simulink model "GA_driveline_Gear_19a"  (R2019a)
settings: Solver=ode23t  StartTime=0.0  StopTime=1  MaxStep=1e-2  RelTol=1e-3  AbsTol=1e-3  EnableMultiTasking=on
StopFcn:
  | GA_plot
libraries: fl_lib x29, nesl_utility x20, sdl_lib x4
CloseFcn:
  | try,close(h1_sdl_gear_backlash),end
  | clear h1_sdl_gear_backlash
  | 
  | 
  | clear simlog_sdl_gear_backlash
Description:
  | Gear with Backlash
settings Model: FPTRunName=Active  ExtModeAutoUpdateStatusClock=off  Creator=MathWorks  LastModifiedBy=JPark
settings SolverCC: AutoScaleAbsTol=off
settings DataIOCC: MaxDataPoints=10000  SaveFormat=Array  SignalLoggingSaveFormat=ModelDataLogs  SaveOutput=off  SignalLogging=off  DSMLogging=off  ReturnWorkspaceOutputs=off  SignalLoggingName=logsout_sdl_gear_backlash
settings OptimizationCC: ExpressionDepthLimit=2147483647  InitFltsAndDblsToZero=on  LifeSpan=inf
settings DebuggingCC: AlgebraicLoopMsg=none  SaveWithParameterizedLinksMsg=none  SignalResolutionControl=TryResolveAllWithWarning  MultiTaskDSMMsg=warning  MultiTaskCondExecSysMsg=none  SigSpecEnsureSampleTimeMsg=none  StateNameClashWarn=warning  SFUnexpectedBacktrackingDiag=warning  SFNoUnconditionalDefaultTransitionDiag=warning  SFExecutionAtInitializationDiag=none  ArithmeticOperatorsInVariantConditions=warning
settings HardwareCC: ProdBitPerPointer=32  ProdBitPerSizeT=32  ProdBitPerPtrDiffT=32  ProdLargestAtomicFloat=None  ProdIntDivRoundTo=Undefined  ProdEndianess=Unspecified  ProdWordSize=32  ProdHWDeviceType=32-bit Generic  TargetBitPerPointer=64  TargetBitPerSizeT=64  TargetBitPerPtrDiffT=64  TargetLongLongMode=on  TargetIntDivRoundTo=Zero  TargetEndianess=LittleEndian  TargetWordSize=64  TargetHWDeviceType=MATLAB Host  ProdEqTarget=off
settings ModelReferenceCC: PropagateSignalLabelsOutOfModel=off
settings SFSimCC: SimUseLocalCustomCode=off
settings RTWCC: Description=Generic Real-Time Target  RTWUseLocalCustomCode=off
settings CodeAppCC: StateflowObjectComments=on
settings GRTTargetCC: TargetLangStandard=C89/C90 (ANSI)  GeneratePreprocessorConditionals=Disable all  CombineOutputUpdateFcns=off  GRTInterface=on
settings ConfigComp: CovMetricSettings=dw  CovHtmlReporting=on  CovSaveCumulativeToWorkspaceVar=on  CovSaveSingleToWorkspaceVar=on  CovShowResultsExplorer=off  CovExternalEMLEnable=off
settings SimscapeCC: SimscapeLogType=all  SimscapeLogSimulationStatistics=on  SimscapeLogName=simlog_sdl_gear_backlash  SimscapeLogLimitData=off  SimscapeLogDataHistory=15000

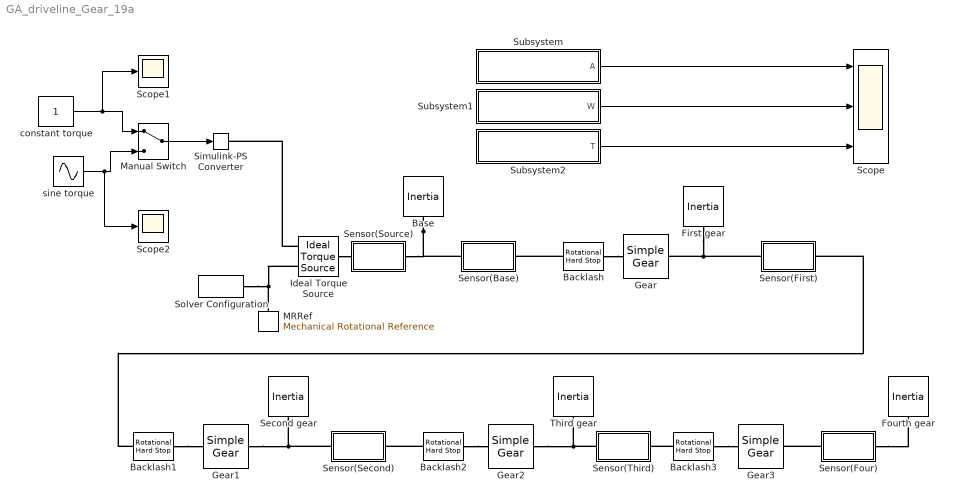
== system GA_driveline_Gear_19a ==
  Backlash{,1..3} (4 alike) : fl_lib/Mechanical/Rotational Elements/Rotational Hard Stop  upper_bnd=0.2 deg  lower_bnd=-0.2 deg  stiff_up=1e+6 N*m/rad  stiff_low=1e+6 N*m/rad  D_up=100 N*m/(rad/s)  D_low=100 N*m/(rad/s)  model=simscape.enum.hardstop.fulldamped  transition=0.001 rad  w_specify=off  w_priority=None  w=0 rad/s  w_nominal_specify=off  w_nominal_unit=rad/s  w_nominal_value=1  t_specify=off  t_priority=None  t=0 N*m  t_nominal_specify=off  t_nominal_unit=N*m  t_nominal_value=1  phi_specify=on  phi_priority=High  phi=0 rad  phi_nominal_specify=off  phi_nominal_unit=rad  phi_nominal_value=1
      settings: SourceProductName=Simscape  SourceProductBaseCode=SS
  Base : fl_lib/Mechanical/Rotational Elements/Inertia  inertia=1 kg*m^2  w_specify=on  w_priority=High  w=0 rad/s  w_nominal_specify=off  w_nominal_unit=rad/s  w_nominal_value=1  t_specify=off  t_priority=None  t=0 N*m  t_nominal_specify=off  t_nominal_unit=N*m  t_nominal_value=1
  First gear : fl_lib/Mechanical/Rotational Elements/Inertia  inertia=1 kg*m^2  w_specify=on  w_priority=High  w=0 rad/s  w_nominal_specify=off  w_nominal_unit=rad/s  w_nominal_value=1  t_specify=off  t_priority=None  t=0 N*m  t_nominal_specify=off  t_nominal_unit=N*m  t_nominal_value=1
  Fourth gear : fl_lib/Mechanical/Rotational Elements/Inertia  inertia=2e-5 kg*m^2  w_specify=on  w_priority=High  w=0 rad/s  w_nominal_specify=off  w_nominal_unit=rad/s  w_nominal_value=1  t_specify=off  t_priority=None  t=0 N*m  t_nominal_specify=off  t_nominal_unit=N*m  t_nominal_value=1
  Gear : sdl_lib/Gears/Simple Gear  ratio=4.5  rotation_direction=1  friction_model=sdl.enum.gear_efficiencies_load.off  T_noload=0.1 N*m  T_nom=5 N*m  efficiency_nom=0.8  efficiency=0.8  mu_visc=[ 0 0 ] N*m/(rad/s)  w_thr=0.01 rad/s  pwr_thr=0.001 W  enable_faults=simscape.enum.onoff.off  efficiency_fault=0.05  external_fault=simscape.enum.onoff.off  temporal_fault=simscape.enum.onoff.off  fault_time=5 s  fault_angles=pi / 12 rad  report_fault=1  temperature_TLU=[ 280 300 320 ] K  load_TLU=[ 1 5 10 ] N*m  efficiency_TLU=[ 0.95 0.9 0.85 ]  efficiency_TLU2=[ 0.85 0.8 0.75; 0.95 0.9 0.85; 0.85 0.8 0.7 ]  thermal_mass=50 J/K  T_init=300 K
      settings: SourceProductName=Simscape Driveline
  Gear1 : sdl_lib/Gears/Simple Gear  ratio=4.5  rotation_direction=1  friction_model=sdl.enum.gear_efficiencies_load.off  T_noload=0.1 N*m  T_nom=5 N*m  efficiency_nom=0.8  efficiency=0.8  mu_visc=[ 0 0 ] N*m/(rad/s)  w_thr=0.01 rad/s  pwr_thr=0.001 W  enable_faults=simscape.enum.onoff.off  efficiency_fault=0.05  external_fault=simscape.enum.onoff.off  temporal_fault=simscape.enum.onoff.off  fault_time=5 s  fault_angles=pi / 12 rad  report_fault=1  temperature_TLU=[ 280 300 320 ] K  load_TLU=[ 1 5 10 ] N*m  efficiency_TLU=[ 0.95 0.9 0.85 ]  efficiency_TLU2=[ 0.85 0.8 0.75; 0.95 0.9 0.85; 0.85 0.8 0.7 ]  thermal_mass=50 J/K  T_init=300 K
      settings: SourceProductName=Simscape Driveline
  Gear2 : sdl_lib/Gears/Simple Gear  ratio=4.5  rotation_direction=1  friction_model=sdl.enum.gear_efficiencies_load.off  T_noload=0.1 N*m  T_nom=5 N*m  efficiency_nom=0.8  efficiency=0.8  mu_visc=[ 0 0 ] N*m/(rad/s)  w_thr=0.01 rad/s  pwr_thr=0.001 W  enable_faults=simscape.enum.onoff.off  efficiency_fault=0.05  external_fault=simscape.enum.onoff.off  temporal_fault=simscape.enum.onoff.off  fault_time=5 s  fault_angles=pi / 12 rad  report_fault=1  temperature_TLU=[ 280 300 320 ] K  load_TLU=[ 1 5 10 ] N*m  efficiency_TLU=[ 0.95 0.9 0.85 ]  efficiency_TLU2=[ 0.85 0.8 0.75; 0.95 0.9 0.85; 0.85 0.8 0.7 ]  thermal_mass=50 J/K  T_init=300 K
      settings: SourceProductName=Simscape Driveline
  Gear3 : sdl_lib/Gears/Simple Gear  ratio=3.1  rotation_direction=1  friction_model=sdl.enum.gear_efficiencies_load.off  T_noload=0.1 N*m  T_nom=5 N*m  efficiency_nom=0.8  efficiency=0.8  mu_visc=[ 0 0 ] N*m/(rad/s)  w_thr=0.01 rad/s  pwr_thr=0.001 W  enable_faults=simscape.enum.onoff.off  efficiency_fault=0.05  external_fault=simscape.enum.onoff.off  temporal_fault=simscape.enum.onoff.off  fault_time=5 s  fault_angles=pi / 12 rad  report_fault=1  temperature_TLU=[ 280 300 320 ] K  load_TLU=[ 1 5 10 ] N*m  efficiency_TLU=[ 0.95 0.9 0.85 ]  efficiency_TLU2=[ 0.85 0.8 0.75; 0.95 0.9 0.85; 0.85 0.8 0.7 ]  thermal_mass=50 J/K  T_init=300 K
      settings: SourceProductName=Simscape Driveline
  Ideal Torque Source : fl_lib/Mechanical/Mechanical Sources/Ideal Torque Source
  MRRef : fl_lib/Mechanical/Rotational Elements/Mechanical Rotational Reference
  Manual Switch : ManualSwitch
  Scope : Scope  NumInputPorts=3
  Scope1 : Scope
  Scope2 : Scope
  Second gear : fl_lib/Mechanical/Rotational Elements/Inertia  inertia=1 kg*m^2  w_specify=on  w_priority=High  w=0 rad/s  w_nominal_specify=off  w_nominal_unit=rad/s  w_nominal_value=1  t_specify=off  t_priority=None  t=0 N*m  t_nominal_specify=off  t_nominal_unit=N*m  t_nominal_value=1
  Sensor(Base) : Subsystem
  Sensor(First) : Subsystem
  Sensor(Four) : Subsystem
  Sensor(Second) : Subsystem
  Sensor(Source) : Subsystem
  Sensor(Third) : Subsystem
  Simulink-PS Converter : nesl_utility/Simulink-PS Converter  PhysicalDomain=network_engine_domain  SubClassName=ps_input  LeftPortType=input  RightPortType=output  PseudoPeriodic=off  Frequencies=[]  NoiseDistribution=none  NoiseParameters=[]  Unit=1  AffineConversion=off  FilteringAndDerivatives=provide  SimscapeFilterOrder=1  InputFilterTimeConstant=0.001  UdotUserProvided=0
  Solver Configuration : nesl_utility/Solver Configuration  PhysicalDomain=network_engine_domain  SubClassName=solver  LeftPortType=input  RightPortType=generic  Tones=[]  Harmonics=[]  SimulateNoise=off  Profile=off  UseLocalSampling=off  EnableSwitchedLinearOptims=on  FrequencyDomain=off  UseCCode=off  RelTol=0.001  AbsTol=1e-06  MinStep=1e-09  ToWorkspace=off  RevertToSquareIcSolve=off  NumHomotopyIterations=100  PhasorMode=off  PhasorModeNumHarmonics=1  DoDC=off  ResidualTolerance=1e-9  UseLocalSolver=off  LocalSolverChoice=NE_PARTITIONING_ADVANCER  LocalSolverSampleTime=0.0001  DoFixedCost=off  MaxNonlinIter=3  MaxModeIter=2  LinearAlgebra=auto  EquationFormulation=NE_TIME_EF  DelaysMemoryBudget=1024  AutomaticFiltering=on  FilteringTimeConstant=0.001  PartitionStorageMethod=EXHAUSTIVE  PartitionMemoryBudget=1024  PartitionMethod=ROBUST
  Subsystem : Subsystem
  Subsystem1 : Subsystem
  Subsystem2 : Subsystem
  Third gear : fl_lib/Mechanical/Rotational Elements/Inertia  inertia=1 kg*m^2  w_specify=on  w_priority=High  w=0 rad/s  w_nominal_specify=off  w_nominal_unit=rad/s  w_nominal_value=1  t_specify=off  t_priority=None  t=0 N*m  t_nominal_specify=off  t_nominal_unit=N*m  t_nominal_value=1
  constant torque : Constant
  sine torque : Sin  Amplitude=100  Frequency=2*pi*1  Phase=1/2*pi  SampleTime=0
  wires:
  constant torque/1 -> Scope1/1, Manual Switch/1
  sine torque/1 -> Scope2/1, Manual Switch/2
  Manual Switch/1 -> Simulink-PS Converter/1
  Subsystem/1(A) -> Scope/1
  Subsystem1/1(W) -> Scope/2
  Subsystem2/1(T) -> Scope/3
  connections:
  Base/LConn1 -- Sensor(Source)/RConn1 -- Sensor(Base)/LConn1
  MRRef/LConn1 -- Ideal Torque Source/RConn2 -- Solver Configuration/RConn1
  Backlash/RConn1 -- Gear/LConn1
  First gear/LConn1 -- Sensor(First)/LConn1 -- Gear/RConn1
  Backlash1/RConn1 -- Gear1/LConn1
  Gear1/RConn1 -- Sensor(Second)/LConn1 -- Second gear/LConn1
  Gear2/RConn1 -- Sensor(Third)/LConn1 -- Third gear/LConn1
  Backlash2/RConn1 -- Gear2/LConn1
  Backlash3/RConn1 -- Gear3/LConn1
  Ideal Torque Source/RConn1 -- Simulink-PS Converter/RConn1
  Backlash/LConn1 -- Sensor(Base)/RConn1
  Backlash1/LConn1 -- Sensor(First)/RConn1
  Backlash2/LConn1 -- Sensor(Second)/RConn1
  Backlash3/LConn1 -- Sensor(Third)/RConn1
  Sensor(Four)/LConn1 -- Gear3/RConn1
  Sensor(Four)/RConn1 -- Fourth gear/LConn1
  Ideal Torque Source/LConn1 -- Sensor(Source)/LConn1

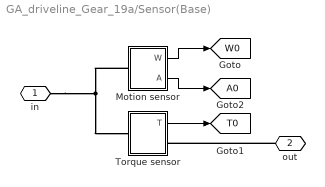
== system GA_driveline_Gear_19a/Sensor(Base) ==
  Motion sensor : Subsystem
  Torque sensor : Subsystem
  in : PMIOPort  Side=Left
  out : PMIOPort  Port=2  Side=Right
  tag scope: A0=global, T0=global, W0=global
  wires:
  Motion sensor/1(W) -> [W0]
  Torque sensor/1(T) -> [T0]
  Motion sensor/2(A) -> [A0]
  connections:
  in/RConn1 -- Motion sensor/LConn1 -- Torque sensor/LConn1
  out/RConn1 -- Torque sensor/RConn1

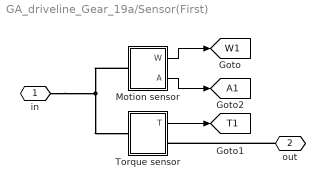
== system GA_driveline_Gear_19a/Sensor(First) ==
  Motion sensor : Subsystem
  Torque sensor : Subsystem
  in : PMIOPort  Side=Left
  out : PMIOPort  Port=2  Side=Right
  tag scope: A1=global, T1=global, W1=global
  wires:
  Motion sensor/1(W) -> [W1]
  Torque sensor/1(T) -> [T1]
  Motion sensor/2(A) -> [A1]
  connections:
  in/RConn1 -- Motion sensor/LConn1 -- Torque sensor/LConn1
  out/RConn1 -- Torque sensor/RConn1

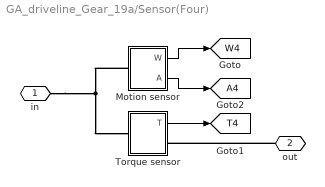
== system GA_driveline_Gear_19a/Sensor(Four) ==
  Motion sensor : Subsystem
  Torque sensor : Subsystem
  in : PMIOPort  Side=Left
  out : PMIOPort  Port=2  Side=Right
  tag scope: A4=global, T4=global, W4=global
  wires:
  Motion sensor/1(W) -> [W4]
  Torque sensor/1(T) -> [T4]
  Motion sensor/2(A) -> [A4]
  connections:
  in/RConn1 -- Motion sensor/LConn1 -- Torque sensor/LConn1
  out/RConn1 -- Torque sensor/RConn1

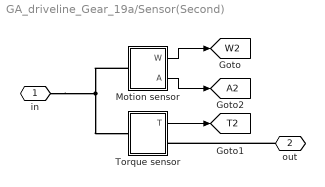
== system GA_driveline_Gear_19a/Sensor(Second) ==
  Motion sensor : Subsystem
  Torque sensor : Subsystem
  in : PMIOPort  Side=Left
  out : PMIOPort  Port=2  Side=Right
  tag scope: A2=global, T2=global, W2=global
  wires:
  Motion sensor/1(W) -> [W2]
  Torque sensor/1(T) -> [T2]
  Motion sensor/2(A) -> [A2]
  connections:
  in/RConn1 -- Motion sensor/LConn1 -- Torque sensor/LConn1
  out/RConn1 -- Torque sensor/RConn1

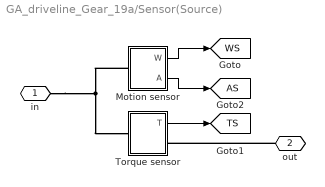
== system GA_driveline_Gear_19a/Sensor(Source) ==
  Motion sensor : Subsystem
  Torque sensor : Subsystem
  in : PMIOPort  Side=Left
  out : PMIOPort  Port=2  Side=Right
  tag scope: AS=global, TS=global, WS=global
  wires:
  Motion sensor/1(W) -> [WS]
  Torque sensor/1(T) -> [TS]
  Motion sensor/2(A) -> [AS]
  connections:
  in/RConn1 -- Motion sensor/LConn1 -- Torque sensor/LConn1
  out/RConn1 -- Torque sensor/RConn1

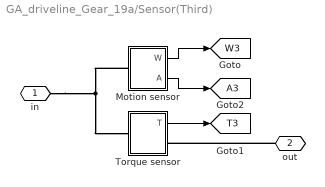
== system GA_driveline_Gear_19a/Sensor(Third) ==
  Motion sensor : Subsystem
  Torque sensor : Subsystem
  in : PMIOPort  Side=Left
  out : PMIOPort  Port=2  Side=Right
  tag scope: A3=global, T3=global, W3=global
  wires:
  Motion sensor/1(W) -> [W3]
  Torque sensor/1(T) -> [T3]
  Motion sensor/2(A) -> [A3]
  connections:
  in/RConn1 -- Motion sensor/LConn1 -- Torque sensor/LConn1
  out/RConn1 -- Torque sensor/RConn1

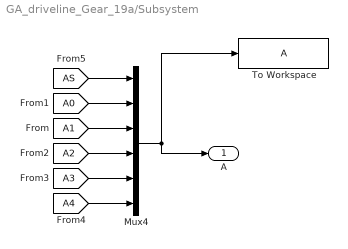
== system GA_driveline_Gear_19a/Subsystem ==
  Mux4 : Mux  Inputs=6
  To Workspace : ToWorkspace  VariableName=A  SaveFormat=Timeseries  SampleTime=-1
  A : Outport
  wires:
  Mux4/1 -> A/1, To Workspace/1
  [AS] -> Mux4/1
  [A0] -> Mux4/2
  [A1] -> Mux4/3
  [A2] -> Mux4/4
  [A3] -> Mux4/5
  [A4] -> Mux4/6

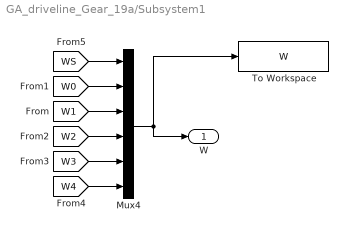
== system GA_driveline_Gear_19a/Subsystem1 ==
  Mux4 : Mux  Inputs=6
  To Workspace : ToWorkspace  VariableName=W  SaveFormat=Timeseries  SampleTime=-1
  W : Outport
  wires:
  Mux4/1 -> W/1, To Workspace/1
  [WS] -> Mux4/1
  [W0] -> Mux4/2
  [W1] -> Mux4/3
  [W2] -> Mux4/4
  [W3] -> Mux4/5
  [W4] -> Mux4/6

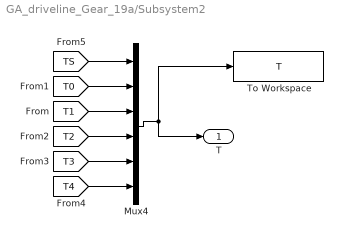
== system GA_driveline_Gear_19a/Subsystem2 ==
  Mux4 : Mux  Inputs=6
  To Workspace : ToWorkspace  VariableName=T  SaveFormat=Timeseries  SampleTime=-1
  T : Outport
  wires:
  Mux4/1 -> T/1, To Workspace/1
  [TS] -> Mux4/1
  [T0] -> Mux4/2
  [T1] -> Mux4/3
  [T2] -> Mux4/4
  [T3] -> Mux4/5
  [T4] -> Mux4/6

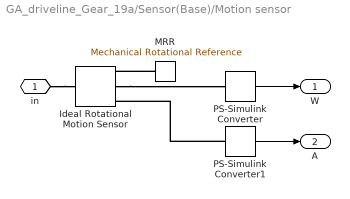
== system GA_driveline_Gear_19a/Sensor(Base)/Motion sensor ==
  Ideal Rotational Motion Sensor : fl_lib/Mechanical/Mechanical Sensors/Ideal Rotational Motion Sensor  offset=0 rad
  MRR : fl_lib/Mechanical/Rotational Elements/Mechanical Rotational Reference
  PS-Simulink Converter : nesl_utility/PS-Simulink Converter  PhysicalDomain=network_engine_domain  SubClassName=ps_output  LeftPortType=input  RightPortType=output  PseudoPeriodic=off  Frequencies=[]  Unit=rad/s  AffineConversion=off
  PS-Simulink Converter1 : nesl_utility/PS-Simulink Converter  PhysicalDomain=network_engine_domain  SubClassName=ps_output  LeftPortType=input  RightPortType=output  PseudoPeriodic=off  Frequencies=[]  Unit=rad  AffineConversion=off
  in : PMIOPort  Side=Left
  W : Outport  VectorParamsAs1DForOutWhenUnconnected=off
  A : Outport  Port=2  VectorParamsAs1DForOutWhenUnconnected=off
  wires:
  PS-Simulink Converter/1 -> W/1
  PS-Simulink Converter1/1 -> A/1
  connections:
  in/RConn1 -- Ideal Rotational Motion Sensor/LConn1
  Ideal Rotational Motion Sensor/RConn2 -- PS-Simulink Converter/LConn1
  MRR/LConn1 -- Ideal Rotational Motion Sensor/RConn1
  PS-Simulink Converter1/LConn1 -- Ideal Rotational Motion Sensor/RConn3

== system GA_driveline_Gear_19a/Sensor(Base)/Torque sensor ==
  PS2S : nesl_utility/PS-Simulink Converter  PhysicalDomain=network_engine_domain  SubClassName=ps_output  LeftPortType=input  RightPortType=output  PseudoPeriodic=off  Frequencies=[]  Unit=N*m  AffineConversion=off
  Torque Sensor : fl_lib/Mechanical/Mechanical Sensors/Ideal Torque Sensor
  B : PMIOPort  Side=Right
  in : PMIOPort  Port=2  Side=Left
  T : Outport  VectorParamsAs1DForOutWhenUnconnected=off
  wires:
  PS2S/1 -> T/1
  connections:
  in/RConn1 -- Torque Sensor/LConn1
  B/RConn1 -- Torque Sensor/RConn1
  Torque Sensor/RConn2 -- PS2S/LConn1

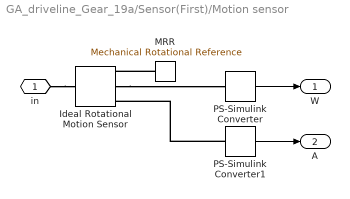
== system GA_driveline_Gear_19a/Sensor(First)/Motion sensor ==
  Ideal Rotational Motion Sensor : fl_lib/Mechanical/Mechanical Sensors/Ideal Rotational Motion Sensor  offset=0 rad
  MRR : fl_lib/Mechanical/Rotational Elements/Mechanical Rotational Reference
  PS-Simulink Converter : nesl_utility/PS-Simulink Converter  PhysicalDomain=network_engine_domain  SubClassName=ps_output  LeftPortType=input  RightPortType=output  PseudoPeriodic=off  Frequencies=[]  Unit=rad/s  AffineConversion=off
  PS-Simulink Converter1 : nesl_utility/PS-Simulink Converter  PhysicalDomain=network_engine_domain  SubClassName=ps_output  LeftPortType=input  RightPortType=output  PseudoPeriodic=off  Frequencies=[]  Unit=rad  AffineConversion=off
  in : PMIOPort  Side=Left
  W : Outport  VectorParamsAs1DForOutWhenUnconnected=off
  A : Outport  Port=2  VectorParamsAs1DForOutWhenUnconnected=off
  wires:
  PS-Simulink Converter/1 -> W/1
  PS-Simulink Converter1/1 -> A/1
  connections:
  in/RConn1 -- Ideal Rotational Motion Sensor/LConn1
  Ideal Rotational Motion Sensor/RConn2 -- PS-Simulink Converter/LConn1
  MRR/LConn1 -- Ideal Rotational Motion Sensor/RConn1
  PS-Simulink Converter1/LConn1 -- Ideal Rotational Motion Sensor/RConn3

== system GA_driveline_Gear_19a/Sensor(First)/Torque sensor ==
  PS2S : nesl_utility/PS-Simulink Converter  PhysicalDomain=network_engine_domain  SubClassName=ps_output  LeftPortType=input  RightPortType=output  PseudoPeriodic=off  Frequencies=[]  Unit=N*m  AffineConversion=off
  Torque Sensor : fl_lib/Mechanical/Mechanical Sensors/Ideal Torque Sensor
  B : PMIOPort  Side=Right
  in : PMIOPort  Port=2  Side=Left
  T : Outport  VectorParamsAs1DForOutWhenUnconnected=off
  wires:
  PS2S/1 -> T/1
  connections:
  in/RConn1 -- Torque Sensor/LConn1
  B/RConn1 -- Torque Sensor/RConn1
  Torque Sensor/RConn2 -- PS2S/LConn1

== system GA_driveline_Gear_19a/Sensor(Four)/Motion sensor ==
  Ideal Rotational Motion Sensor : fl_lib/Mechanical/Mechanical Sensors/Ideal Rotational Motion Sensor  offset=0 rad
  MRR : fl_lib/Mechanical/Rotational Elements/Mechanical Rotational Reference
  PS-Simulink Converter : nesl_utility/PS-Simulink Converter  PhysicalDomain=network_engine_domain  SubClassName=ps_output  LeftPortType=input  RightPortType=output  PseudoPeriodic=off  Frequencies=[]  Unit=rad/s  AffineConversion=off
  PS-Simulink Converter1 : nesl_utility/PS-Simulink Converter  PhysicalDomain=network_engine_domain  SubClassName=ps_output  LeftPortType=input  RightPortType=output  PseudoPeriodic=off  Frequencies=[]  Unit=rad  AffineConversion=off
  in : PMIOPort  Side=Left
  W : Outport  VectorParamsAs1DForOutWhenUnconnected=off
  A : Outport  Port=2  VectorParamsAs1DForOutWhenUnconnected=off
  wires:
  PS-Simulink Converter/1 -> W/1
  PS-Simulink Converter1/1 -> A/1
  connections:
  in/RConn1 -- Ideal Rotational Motion Sensor/LConn1
  Ideal Rotational Motion Sensor/RConn2 -- PS-Simulink Converter/LConn1
  MRR/LConn1 -- Ideal Rotational Motion Sensor/RConn1
  PS-Simulink Converter1/LConn1 -- Ideal Rotational Motion Sensor/RConn3

== system GA_driveline_Gear_19a/Sensor(Four)/Torque sensor ==
  PS2S : nesl_utility/PS-Simulink Converter  PhysicalDomain=network_engine_domain  SubClassName=ps_output  LeftPortType=input  RightPortType=output  PseudoPeriodic=off  Frequencies=[]  Unit=N*m  AffineConversion=off
  Torque Sensor : fl_lib/Mechanical/Mechanical Sensors/Ideal Torque Sensor
  B : PMIOPort  Side=Right
  in : PMIOPort  Port=2  Side=Left
  T : Outport  VectorParamsAs1DForOutWhenUnconnected=off
  wires:
  PS2S/1 -> T/1
  connections:
  in/RConn1 -- Torque Sensor/LConn1
  B/RConn1 -- Torque Sensor/RConn1
  Torque Sensor/RConn2 -- PS2S/LConn1

== system GA_driveline_Gear_19a/Sensor(Second)/Motion sensor ==
  Ideal Rotational Motion Sensor : fl_lib/Mechanical/Mechanical Sensors/Ideal Rotational Motion Sensor  offset=0 rad
  MRR : fl_lib/Mechanical/Rotational Elements/Mechanical Rotational Reference
  PS-Simulink Converter : nesl_utility/PS-Simulink Converter  PhysicalDomain=network_engine_domain  SubClassName=ps_output  LeftPortType=input  RightPortType=output  PseudoPeriodic=off  Frequencies=[]  Unit=rad/s  AffineConversion=off
  PS-Simulink Converter1 : nesl_utility/PS-Simulink Converter  PhysicalDomain=network_engine_domain  SubClassName=ps_output  LeftPortType=input  RightPortType=output  PseudoPeriodic=off  Frequencies=[]  Unit=rad  AffineConversion=off
  in : PMIOPort  Side=Left
  W : Outport  VectorParamsAs1DForOutWhenUnconnected=off
  A : Outport  Port=2  VectorParamsAs1DForOutWhenUnconnected=off
  wires:
  PS-Simulink Converter/1 -> W/1
  PS-Simulink Converter1/1 -> A/1
  connections:
  in/RConn1 -- Ideal Rotational Motion Sensor/LConn1
  Ideal Rotational Motion Sensor/RConn2 -- PS-Simulink Converter/LConn1
  MRR/LConn1 -- Ideal Rotational Motion Sensor/RConn1
  PS-Simulink Converter1/LConn1 -- Ideal Rotational Motion Sensor/RConn3

== system GA_driveline_Gear_19a/Sensor(Second)/Torque sensor ==
  PS2S : nesl_utility/PS-Simulink Converter  PhysicalDomain=network_engine_domain  SubClassName=ps_output  LeftPortType=input  RightPortType=output  PseudoPeriodic=off  Frequencies=[]  Unit=N*m  AffineConversion=off
  Torque Sensor : fl_lib/Mechanical/Mechanical Sensors/Ideal Torque Sensor
  B : PMIOPort  Side=Right
  in : PMIOPort  Port=2  Side=Left
  T : Outport  VectorParamsAs1DForOutWhenUnconnected=off
  wires:
  PS2S/1 -> T/1
  connections:
  in/RConn1 -- Torque Sensor/LConn1
  B/RConn1 -- Torque Sensor/RConn1
  Torque Sensor/RConn2 -- PS2S/LConn1

== system GA_driveline_Gear_19a/Sensor(Source)/Motion sensor ==
  Ideal Rotational Motion Sensor : fl_lib/Mechanical/Mechanical Sensors/Ideal Rotational Motion Sensor  offset=0 rad
  MRR : fl_lib/Mechanical/Rotational Elements/Mechanical Rotational Reference
  PS-Simulink Converter : nesl_utility/PS-Simulink Converter  PhysicalDomain=network_engine_domain  SubClassName=ps_output  LeftPortType=input  RightPortType=output  PseudoPeriodic=off  Frequencies=[]  Unit=rad/s  AffineConversion=off
  PS-Simulink Converter1 : nesl_utility/PS-Simulink Converter  PhysicalDomain=network_engine_domain  SubClassName=ps_output  LeftPortType=input  RightPortType=output  PseudoPeriodic=off  Frequencies=[]  Unit=rad  AffineConversion=off
  in : PMIOPort  Side=Left
  W : Outport  VectorParamsAs1DForOutWhenUnconnected=off
  A : Outport  Port=2  VectorParamsAs1DForOutWhenUnconnected=off
  wires:
  PS-Simulink Converter/1 -> W/1
  PS-Simulink Converter1/1 -> A/1
  connections:
  in/RConn1 -- Ideal Rotational Motion Sensor/LConn1
  Ideal Rotational Motion Sensor/RConn2 -- PS-Simulink Converter/LConn1
  MRR/LConn1 -- Ideal Rotational Motion Sensor/RConn1
  PS-Simulink Converter1/LConn1 -- Ideal Rotational Motion Sensor/RConn3

== system GA_driveline_Gear_19a/Sensor(Source)/Torque sensor ==
  PS2S : nesl_utility/PS-Simulink Converter  PhysicalDomain=network_engine_domain  SubClassName=ps_output  LeftPortType=input  RightPortType=output  PseudoPeriodic=off  Frequencies=[]  Unit=N*m  AffineConversion=off
  Torque Sensor : fl_lib/Mechanical/Mechanical Sensors/Ideal Torque Sensor
  B : PMIOPort  Side=Right
  in : PMIOPort  Port=2  Side=Left
  T : Outport  VectorParamsAs1DForOutWhenUnconnected=off
  wires:
  PS2S/1 -> T/1
  connections:
  in/RConn1 -- Torque Sensor/LConn1
  B/RConn1 -- Torque Sensor/RConn1
  Torque Sensor/RConn2 -- PS2S/LConn1

== system GA_driveline_Gear_19a/Sensor(Third)/Motion sensor ==
  Ideal Rotational Motion Sensor : fl_lib/Mechanical/Mechanical Sensors/Ideal Rotational Motion Sensor  offset=0 rad
  MRR : fl_lib/Mechanical/Rotational Elements/Mechanical Rotational Reference
  PS-Simulink Converter : nesl_utility/PS-Simulink Converter  PhysicalDomain=network_engine_domain  SubClassName=ps_output  LeftPortType=input  RightPortType=output  PseudoPeriodic=off  Frequencies=[]  Unit=rad/s  AffineConversion=off
  PS-Simulink Converter1 : nesl_utility/PS-Simulink Converter  PhysicalDomain=network_engine_domain  SubClassName=ps_output  LeftPortType=input  RightPortType=output  PseudoPeriodic=off  Frequencies=[]  Unit=rad  AffineConversion=off
  in : PMIOPort  Side=Left
  W : Outport  VectorParamsAs1DForOutWhenUnconnected=off
  A : Outport  Port=2  VectorParamsAs1DForOutWhenUnconnected=off
  wires:
  PS-Simulink Converter/1 -> W/1
  PS-Simulink Converter1/1 -> A/1
  connections:
  in/RConn1 -- Ideal Rotational Motion Sensor/LConn1
  Ideal Rotational Motion Sensor/RConn2 -- PS-Simulink Converter/LConn1
  MRR/LConn1 -- Ideal Rotational Motion Sensor/RConn1
  PS-Simulink Converter1/LConn1 -- Ideal Rotational Motion Sensor/RConn3

== system GA_driveline_Gear_19a/Sensor(Third)/Torque sensor ==
  PS2S : nesl_utility/PS-Simulink Converter  PhysicalDomain=network_engine_domain  SubClassName=ps_output  LeftPortType=input  RightPortType=output  PseudoPeriodic=off  Frequencies=[]  Unit=N*m  AffineConversion=off
  Torque Sensor : fl_lib/Mechanical/Mechanical Sensors/Ideal Torque Sensor
  B : PMIOPort  Side=Right
  in : PMIOPort  Port=2  Side=Left
  T : Outport  VectorParamsAs1DForOutWhenUnconnected=off
  wires:
  PS2S/1 -> T/1
  connections:
  in/RConn1 -- Torque Sensor/LConn1
  B/RConn1 -- Torque Sensor/RConn1
  Torque Sensor/RConn2 -- PS2S/LConn1
